simulink model "Q8_W1"  (R2020b)
settings: Solver=VariableStepAuto  StartTime=0.0  StopTime=10.0  RelTol=1e-3
settings Model: EnablePacing=on  PacingRate=0.200000  Creator=hp  LastModifiedBy=hp

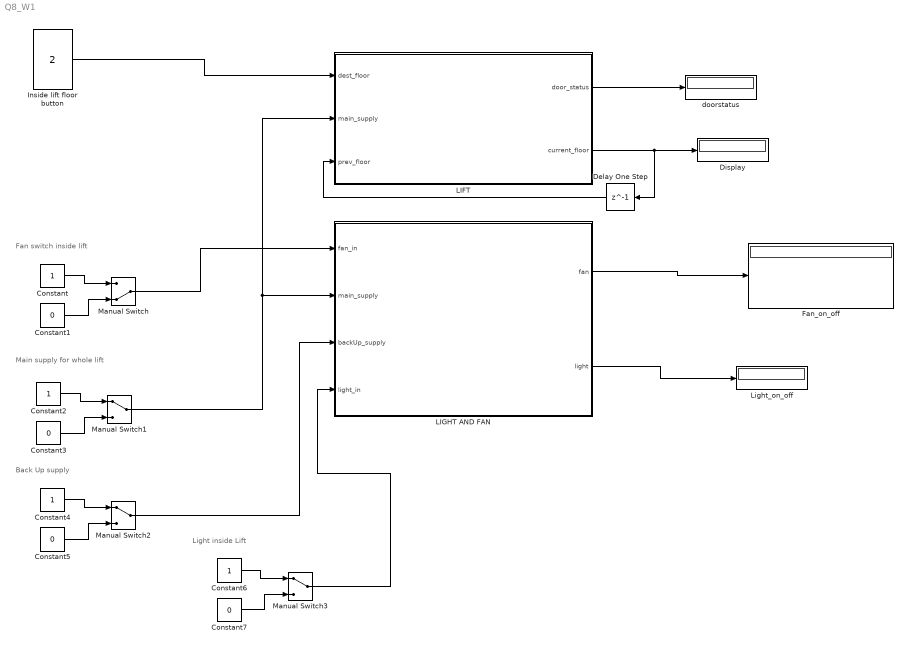
== system Q8_W1 ==
  note: Fan switch inside lift
  note: Main supply for whole lift
  note: Back Up supply
  note: Light inside Lift
  Constant{,2,4,6} (4 alike) : Constant
  Constant{1,3,5,7} (4 alike) : Constant  Value=0
  Delay One Step : Delay  DelayLength=1
  Display : Display
  Fan_on_off : Display
  Inside lift floor button : Constant  Value=2
  LIFT : Stateflow chart  TreatAsAtomicUnit=on
  LIGHT AND FAN : Stateflow chart  TreatAsAtomicUnit=on
  Light_on_off : Display
  Manual Switch : ManualSwitch  CurrentSetting=0
  Manual Switch1 : ManualSwitch
  Manual Switch2 : ManualSwitch
  Manual Switch3 : ManualSwitch
  doorstatus : Display
  wires:
  Constant/1 -> Manual Switch/1
  Constant1/1 -> Manual Switch/2
  Constant3/1 -> Manual Switch1/2
  Constant2/1 -> Manual Switch1/1
  LIGHT AND FAN/1(fan) -> Fan_on_off/1
  Manual Switch/1 -> LIGHT AND FAN/1(fan_in)
  Manual Switch1/1 -> LIFT/2(main_supply), LIGHT AND FAN/2(main_supply)
  Manual Switch2/1 -> LIGHT AND FAN/3(backUp_supply)
  Constant4/1 -> Manual Switch2/1
  Constant5/1 -> Manual Switch2/2
  Manual Switch3/1 -> LIGHT AND FAN/4(light_in)
  Constant6/1 -> Manual Switch3/1
  Constant7/1 -> Manual Switch3/2
  LIGHT AND FAN/2(light) -> Light_on_off/1
  Inside lift floor button/1 -> LIFT/1(dest_floor)
  LIFT/1(door_status) -> doorstatus/1
  LIFT/2(current_floor) -> Delay One Step/1, Display/1
  Delay One Step/1 -> LIFT/3(prev_floor)

== stateflow chart Q8_W1/LIGHT AND FAN ==
  state Fan_light [parallel]
    settings: executionOrder=1
    state FanStatus [parallel]
      settings: executionOrder=2
      (default) -> (junction 18) : {fan=f(fan_in,main_supply)}
    state LightStatus [parallel]
      settings: executionOrder=1
      (default) -> (junction 23) : {light=L(light_in,main_supply,backUp_supply)}
  data: fan_in1 function_input double; main_supply1 function_input double; fan1 function_output double; light_in1 function_input; main_supply1 function_input; backUp_supply1 function_input; light1 function_output; fan output; fan_in input; main_supply input; backUp_supply input; light_in input; light output
  function fan1 = f(fan_in1, main_supply1):
    | function fan1 = f(fan_in1, main_supply1)
    | 
    | aVarTruthTableCondition_1 = false;
    | aVarTruthTableCondition_2 = false;
    | 
    | 
    | % Fan switch from inside On
    | 
    | aVarTruthTableCondition_1 = logical(fan_in1==1);
    | 
    | % Fan switch from outside On
    | 
    | aVarTruthTableCondition_2 = logical(main_supply1==1);
    | 
    | if (aVarTruthTableCondition_1 && aVarTruthTableCondition_2)
    |     A1();
    | elseif (aVarTruthTableCondition_1 && ~aVarTruthTableCondition_2)
    |     A2();
    | elseif (~aVarTruthTableCondition_1 && aVarTruthTableCondition_2)
    |     A3();
    | else % Default
    |     A4();
    | end
    | 
    | function A1()
    | 
    | % fan is On
    | 
    | fan1=1
    | 
    | function A2()
    | 
    | % fan is Off
    | 
    | fan1=0
    | 
    | function A3()
    | 
    | % Fan is Off
    | 
    | fan1=0
    | 
    | function A4()
    | 
    | % Fan is Off
    | 
    | fan1=0
  function light1=L(light_in1,main_supply1,backUp_supply1):
    | function light1=L(light_in1,main_supply1,backUp_supply1)
    | 
    | aVarTruthTableCondition_1 = false;
    | aVarTruthTableCondition_2 = false;
    | aVarTruthTableCondition_3 = false;
    | 
    | 
    | % Condition #1
    | aVarTruthTableCondition_1 = logical(light_in1==1);
    | 
    | % Condition #2
    | aVarTruthTableCondition_2 = logical(main_supply1==1);
    | 
    | % Condition #3
    | aVarTruthTableCondition_3 = logical(backUp_supply1==1);
    | 
    | if (~aVarTruthTableCondition_1 && aVarTruthTableCondition_2 && aVarTruthTableCondition_3)
    |     B1();
    | elseif (~aVarTruthTableCondition_1 && ~aVarTruthTableCondition_2 && aVarTruthTableCondition_3)
    |     B1();
    | elseif (aVarTruthTableCondition_1 && aVarTruthTableCondition_2 && ~aVarTruthTableCondition_3)
    |     B2();
    | elseif (aVarTruthTableCondition_1 && ~aVarTruthTableCondition_2 && ~aVarTruthTableCondition_3)
    |     B3();
    | elseif (~aVarTruthTableCondition_1 && ~aVarTruthTableCondition_2 && ~aVarTruthTableCondition_3)
    |     B3();
    | elseif (aVarTruthTableCondition_1 && ~aVarTruthTableCondition_2 && aVarTruthTableCondition_3)
    |     B4();
    | elseif (~aVarTruthTableCondition_1 && aVarTruthTableCondition_2 && ~aVarTruthTableCondition_3)
    |     B1();
    | else % Default
    |     B4();
    | end
    | 
    | function B2()
    | 
    | 
    | 
    | light1=1;
    | 
    | function B3()
    | 
    | 
    | 
    | light1=0;
    | 
    | function B4()
    | 
    | 
    | 
    | light1=1;
    | 
    | function B1()
    | 
    | 
    | 
    | light1=0;

== stateflow chart Q8_W1/LIFT ==
  state moving_down
    current_floor=current_floor-1;
  state moving_up
    current_floor=current_floor+1;
  state floor_status
  state LIFT_OFF
    current_floor=prev_floor;
    delay=0;
  state Doors
    (default) -> (junction 11)
    (junction 11) -> (junction 12) [order 1] : [main_supply==0]
    (junction 12) -> (junction 14) : {delay=10;}
    (junction 11) -> (junction 13) [order 2] : {delay=3;}
    (junction 14) -> (junction 13)
    (junction 13) -> (junction 15)
    (junction 15) -> (junction 43)
    (junction 43) -> (junction 45)
    (junction 45) -> (junction 44) [order 1] : [delay>0]
    (junction 44) -> (junction 46) : {delay=delay-1;}
    (junction 45) -> (junction 47) [order 2]
    (junction 46) -> (junction 45)
  moving_up -> moving_up [order 1] : [dest_floor~=current_floor]
  moving_down -> floor_status : [dest_floor==current_floor]{floor_reached=1;}
  floor_status -> moving_down [order 2] : [dest_floor<current_floor]{floor_reached=0;}
  floor_status -> moving_up [order 3] : [dest_floor>current_floor]{floor_reached=0;}
  moving_up -> floor_status [order 2] : [dest_floor==current_floor]{floor_reached=1;}
  LIFT_OFF -> floor_status [order 1] : [(current_floor~=dest_floor) && (main_supply==1)]{floor_reached=0;}
  floor_status -> Doors [order 1] : [floor_reached==1]{door_status=1;}
  (default) -> LIFT_OFF
  LIFT_OFF -> Doors [order 2] : [main_supply==0]{door_status=1;}
  Doors -> LIFT_OFF : [(main_supply==1)&&(delay==0)]{door_status=0}
  data: delay local; dest_floor input; main_supply input; door_status output; floor_reached local; current_floor output; prev_floor input
